simulink model "thirdweek_second"  (R2020a)
settings: Solver=FixedStepDiscrete  StartTime=0.0  StopTime=100  FixedStep=0.1  RelTol=1e-3  EnableMultiTasking=on
undefined symbols (not defined in the file): DiscIntNeverNeededParam
libraries: simulink x1
settings Model: Creator=Admin  LastModifiedBy=Admin

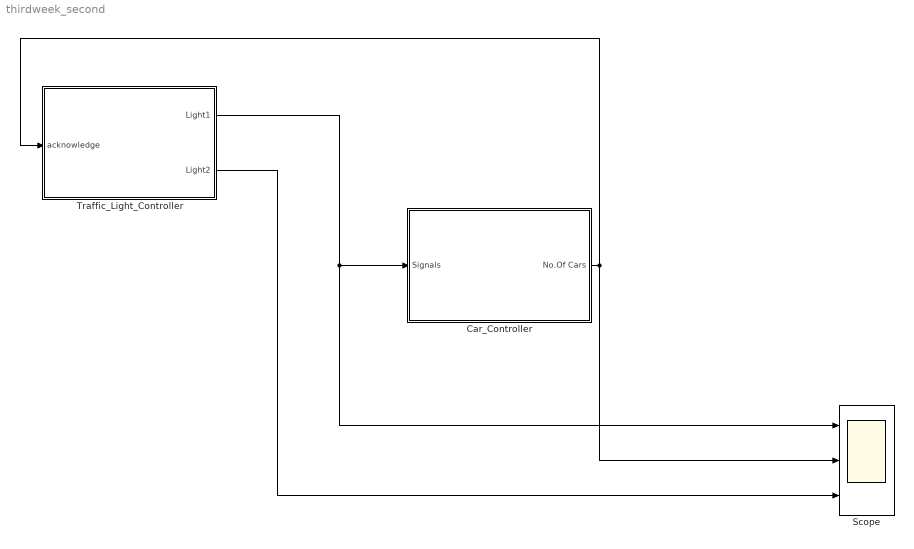
== system thirdweek_second ==
  Car_Controller : Subsystem
  Scope : Scope  NumInputPorts=3
  Traffic_Light_Controller : Stateflow chart  TreatAsAtomicUnit=on
  wires:
  Car_Controller/1(No.Of Cars) -> Traffic_Light_Controller/1(acknowledge), Scope/2
  Traffic_Light_Controller/1(Light1) -> Scope/1, Car_Controller/1(Signals)
  Traffic_Light_Controller/2(Light2) -> Scope/3

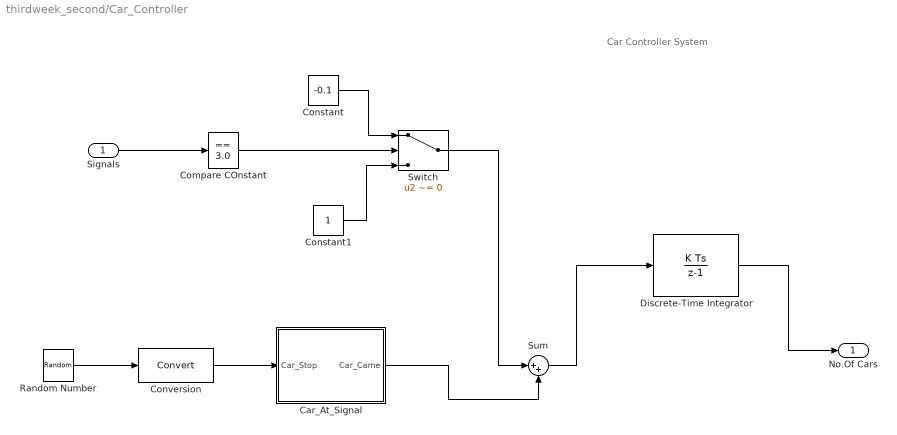
== system thirdweek_second/Car_Controller ==
  note: Car Controller System
  Signals : Inport
  Car_At_Signal : Stateflow chart  TreatAsAtomicUnit=on
  Compare COnstant : simulink/Logic and Bit Operations/Compare To Constant  relop===  const=3.0  OutDataTypeStr=boolean
  Constant : Constant  Value=-0.1
  Constant1 : Constant
  Conversion : DataTypeConversion
  "Discrete-Time Integrator " : DiscreteIntegrator  SampleTime=-1  ICPrevOutput=DiscIntNeverNeededParam  ICPrevScaledInput=DiscIntNeverNeededParam
  Random Number : UniformRandomNumber  Minimum=0  Maximum=150  Seed=150745  SampleTime=0.1
  Sum : Sum  Inputs=|++
  "Switch " : Switch  Criteria=u2 ~= 0
  No.Of Cars : Outport
  wires:
  Conversion/1 -> Car_At_Signal/1(Car_Stop)
  Random Number/1 -> Conversion/1
  "Switch "/1 -> Sum/1
  Constant/1 -> "Switch "/1
  Constant1/1 -> "Switch "/3
  Compare COnstant/1 -> "Switch "/2
  "Discrete-Time Integrator "/1 -> No.Of Cars/1
  Signals/1 -> Compare COnstant/1
  Car_At_Signal/1(Car_Came) -> Sum/2
  Sum/1 -> "Discrete-Time Integrator "/1

== stateflow chart thirdweek_second/Traffic_Light_Controller ==
  state Stop_State
    Light1=Red;
    Light2=Green;
  state Go_To_STop_State
    Light1=Yellow;
    Light2=Red;
  state StopForTraffic_State
    Light1=Red;
    Light2=Green;
  state Ready_To_Go
    Light1=Red;
    Light2=Yellow;
  state Go
    Light1=Green;
    Light2=Red;
  (default) -> Stop_State
  Go_To_STop_State -> Stop_State : after(3,tick)
  Go -> Go_To_STop_State : after(10,tick)
  Stop_State -> StopForTraffic_State : after(20,tick)
  StopForTraffic_State -> Ready_To_Go : [acknowledge]
  Ready_To_Go -> Go : after(3,tick)
  data: acknowledge input; Light1 output; Light2 output; Green constant double =2; Red constant double =1; Yellow constant double =3

== stateflow chart thirdweek_second/Car_Controller/Car_At_Signal ==
  (default) -> (junction 1) : {Car_Came=Car_Stop>90}
  data: Car_Came output; Car_Stop input
